simulink model "MultiSynapseTest_IaF"  (R2020b)
settings: Solver=VariableStepAuto  StartTime=0.0  StopTime=1.0  RelTol=1e-3
libraries: NeuroModelerLibrary x21
settings Model: Creator=Александра  LastModifiedBy=Александра

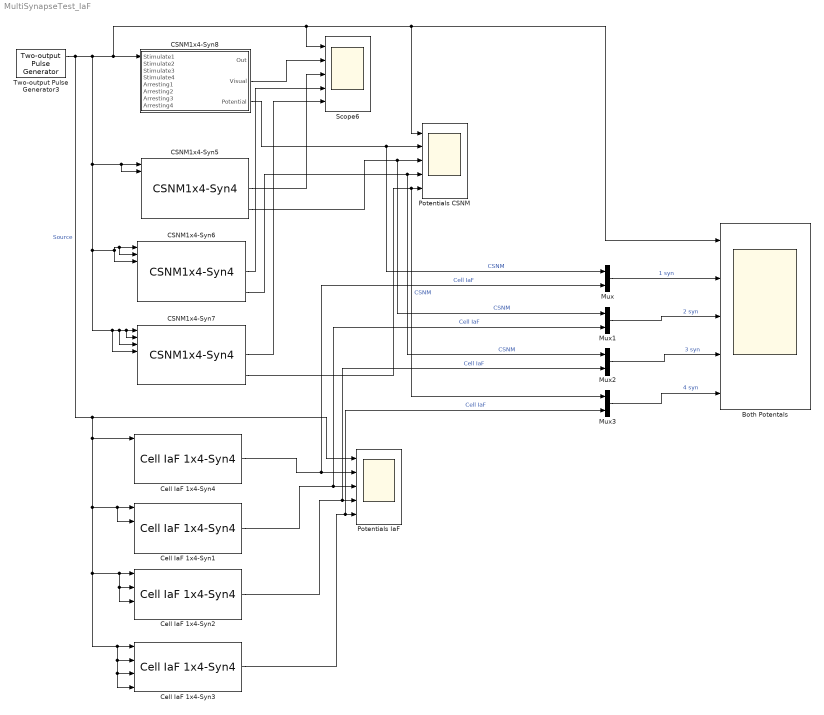
== system MultiSynapseTest_IaF ==
  Both Potentals : Scope  NumInputPorts=5
  CSNM1x4-Syn5 : NeuroModelerLibrary/Sized Cells/CSNM1x4-Syn4  SystemSampleTime=-1  VariantActivationTime=update diagram  Latency=0  AutoFrameSizeCalculation=off
  CSNM1x4-Syn6 : NeuroModelerLibrary/Sized Cells/CSNM1x4-Syn4  SystemSampleTime=-1  VariantActivationTime=update diagram  Latency=0  AutoFrameSizeCalculation=off
  CSNM1x4-Syn7 : NeuroModelerLibrary/Sized Cells/CSNM1x4-Syn4  SystemSampleTime=-1  VariantActivationTime=update diagram  Latency=0  AutoFrameSizeCalculation=off
  CSNM1x4-Syn8 : Subsystem  AncestorBlock=NeuroModelerLibrary/Sized Cells/CSNM1x4-Syn4
  Cell IaF 1x4-Syn{1..4} (4 alike) : NeuroModelerLibrary/Sized Cells/Cell IaF 1x4-Syn4  SystemSampleTime=-1  VariantActivationTime=update diagram  Latency=0  AutoFrameSizeCalculation=off
  Mux{,1..3} (4 alike) : Mux  Inputs=2
  Potentials CSNM : Scope  NumInputPorts=5
  Potentials IaF : Scope  NumInputPorts=5
  Scope6 : Scope  NumInputPorts=5
  Two-output Pulse Generator3 : NeuroModelerLibrary/Support/Two-output Pulse Generator  A=1  P1=200  P2=200  PW=1  ST=0.001  OOn1=0.5  OOff1=0.6  OOn2=0.8  OOff2=0.9
  wires:
  CSNM1x4-Syn7/3 -> Mux3/1, Potentials CSNM/5  "CSNM"
  CSNM1x4-Syn8/3(Potential) -> Mux/1, Potentials CSNM/2  "CSNM"
  CSNM1x4-Syn6/3 -> Mux2/1, Potentials CSNM/4  "CSNM"
  CSNM1x4-Syn6/2 -> Scope6/4
  CSNM1x4-Syn8/2(Visual) -> Scope6/2
  CSNM1x4-Syn7/2 -> Scope6/5
  CSNM1x4-Syn5/2 -> Scope6/3
  CSNM1x4-Syn5/3 -> Mux1/1, Potentials CSNM/3  "CSNM"
  Cell IaF 1x4-Syn4/1 -> Mux/2, Potentials IaF/2  "Cell IaF"
  Cell IaF 1x4-Syn1/1 -> Potentials IaF/3, Mux1/2  "Cell IaF"
  Cell IaF 1x4-Syn2/1 -> Potentials IaF/4, Mux2/2  "Cell IaF"
  Cell IaF 1x4-Syn3/1 -> Mux3/2, Potentials IaF/5  "Cell IaF"
  Two-output Pulse Generator3/1 -> Potentials CSNM/1, Both Potentals/1, Scope6/1, CSNM1x4-Syn8/1(Stimulate1), CSNM1x4-Syn5/1, CSNM1x4-Syn5/2, CSNM1x4-Syn6/3, CSNM1x4-Syn6/1, CSNM1x4-Syn6/2, CSNM1x4-Syn7/4, CSNM1x4-Syn7/3, CSNM1x4-Syn7/2, CSNM1x4-Syn7/1, Cell IaF 1x4-Syn4/1, Cell IaF 1x4-Syn1/1, Cell IaF 1x4-Syn1/2, Cell IaF 1x4-Syn3/1, Cell IaF 1x4-Syn3/2, Cell IaF 1x4-Syn3/4, Cell IaF 1x4-Syn3/3, Cell IaF 1x4-Syn2/1, Cell IaF 1x4-Syn2/3, Cell IaF 1x4-Syn2/2, Potentials IaF/1  "Source"
  Mux/1 -> Both Potentals/2  "1 syn"
  Mux1/1 -> Both Potentals/3  "2 syn"
  Mux2/1 -> Both Potentals/4  "3 syn"
  Mux3/1 -> Both Potentals/5  "4 syn"

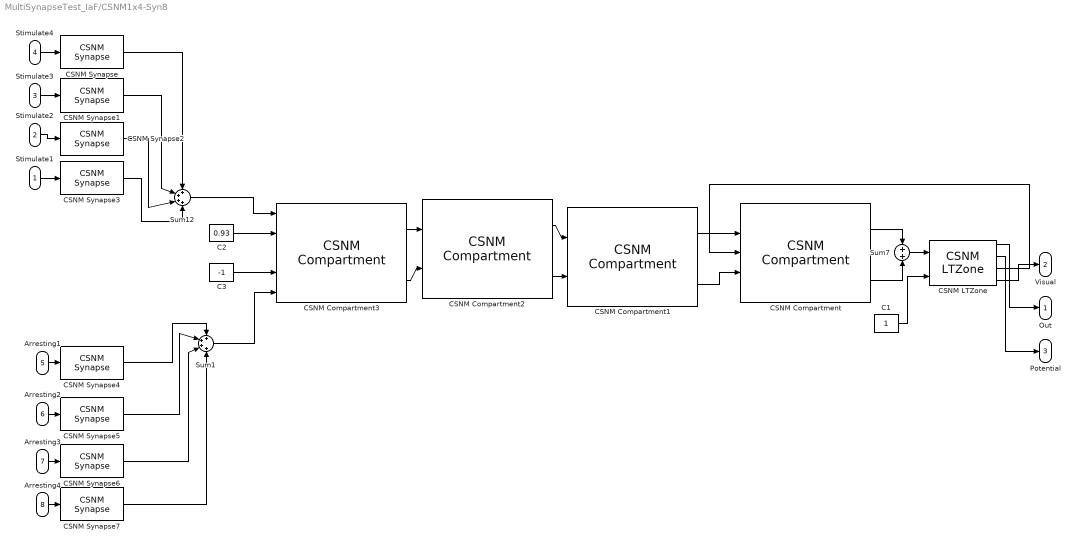
== system MultiSynapseTest_IaF/CSNM1x4-Syn8 ==
  Stimulate1 : Inport
  Stimulate2 : Inport  Port=2
  Stimulate3 : Inport  Port=3
  Stimulate4 : Inport  Port=4
  Arresting1 : Inport  Port=5
  Arresting2 : Inport  Port=6
  Arresting3 : Inport  Port=7
  Arresting4 : Inport  Port=8
  C1 : Constant
  C2 : Constant  Value=0.93
  C3 : Constant  Value=-1
  CSNM Compartment{,1..3} (4 alike) : NeuroModelerLibrary/Neuron Elements/CSNM Compartment  ACm=1e-9  ARm=1e7  ECm=1e-9  ERm=1e7  ARFm=1e7  ERFm=1e7  U0=-0.070  sign=-1
  CSNM LTZone : NeuroModelerLibrary/Neuron Elements/CSNM LTZone  NM=1  FB=2  T=-0.055  switchOff=-0.1
  CSNM Synapse{,1..7} (8 alike) : NeuroModelerLibrary/Neuron Elements/CSNM Synapse  SecretionTC=0.001  DecompositionTC=0.005  UseKsi=off  Rs=2e7  ksi=1  U0=-0.070  Weight=1  sign=off
  Sum1 : Sum  Inputs=++++  InputSameDT=on  SaturateOnIntegerOverflow=on  OutDataTypeStr=Inherit: Same as first input
  Sum12 : Sum  Inputs=++++  InputSameDT=on  SaturateOnIntegerOverflow=on  OutDataTypeStr=Inherit: Same as first input
  Sum7 : Sum  InputSameDT=on  SaturateOnIntegerOverflow=on  OutDataTypeStr=Inherit: Same as first input
  Out : Outport  VectorParamsAs1DForOutWhenUnconnected=off
  Visual : Outport  Port=2  VectorParamsAs1DForOutWhenUnconnected=off
  Potential : Outport  Port=3  VectorParamsAs1DForOutWhenUnconnected=off
  wires:
  Sum12/1 -> CSNM Compartment3/1
  Sum1/1 -> CSNM Compartment3/5
  CSNM LTZone/2 -> Potential/1
  CSNM Compartment/2 -> Sum7/2
  CSNM Compartment/1 -> Sum7/1
  CSNM LTZone/3 -> CSNM Compartment/3
  Sum7/1 -> CSNM LTZone/1
  CSNM Compartment1/2 -> CSNM Compartment/4
  CSNM Compartment1/1 -> CSNM Compartment/2
  Arresting1/1 -> CSNM Synapse4/1
  Stimulate1/1 -> CSNM Synapse3/1
  C1/1 -> CSNM LTZone/2
  CSNM LTZone/1 -> Out/1
  CSNM LTZone/4 -> Visual/1
  CSNM Compartment2/1 -> CSNM Compartment1/2
  CSNM Compartment2/2 -> CSNM Compartment1/4
  CSNM Compartment3/1 -> CSNM Compartment2/2
  CSNM Compartment3/2 -> CSNM Compartment2/4
  CSNM Synapse4/1 -> Sum1/1
  C3/1 -> CSNM Compartment3/4
  C2/1 -> CSNM Compartment3/2
  CSNM Synapse3/1 -> Sum12/4
  CSNM Synapse2/1 -> Sum12/3
  Stimulate2/1 -> CSNM Synapse2/1
  CSNM Synapse1/1 -> Sum12/2
  Stimulate3/1 -> CSNM Synapse1/1
  CSNM Synapse/1 -> Sum12/1
  Stimulate4/1 -> CSNM Synapse/1
  Arresting2/1 -> CSNM Synapse5/1
  CSNM Synapse5/1 -> Sum1/2
  Arresting3/1 -> CSNM Synapse6/1
  CSNM Synapse6/1 -> Sum1/3
  Arresting4/1 -> CSNM Synapse7/1
  CSNM Synapse7/1 -> Sum1/4
